simulink model "task_1_scheme"  (R2024a)
settings: Solver=FixedStepAuto  StartTime=0.0  StopTime=5.0  FixedStep=1e-6  RelTol=1e-3
settings Model: Creator=alexe  LastModifiedBy=alexe

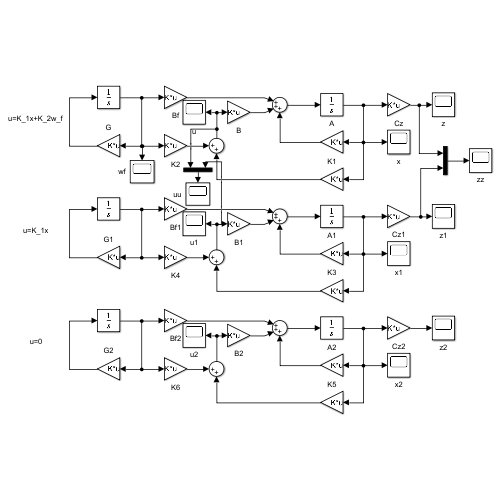
[thumbnail: Simulink's stored preview of the top-level diagram]
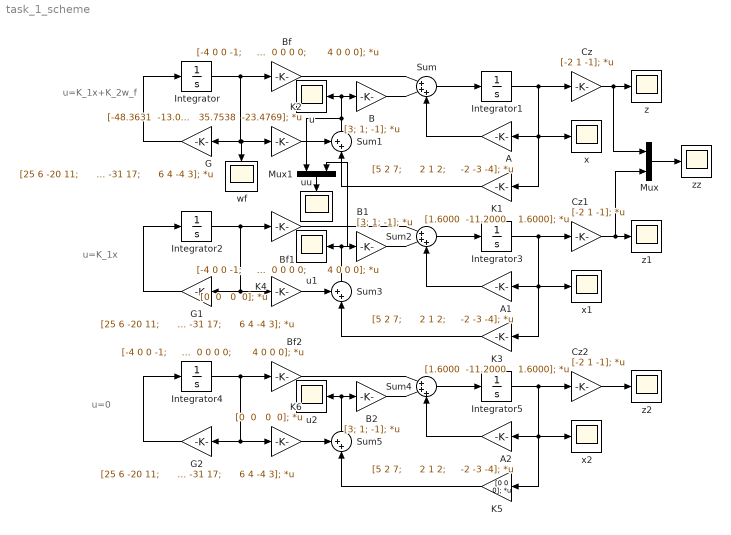
== system task_1_scheme ==
  note: u=K_1x+K_2w_f
  note: u=0
  note: u=K_1x
  A : Gain  Gain=|  Multiplication=Matrix(K*u)
      | [5 2 7;
      |      2 1 2;
      |     -2 -3 -4];
  A1 : Gain  Gain=|  Multiplication=Matrix(K*u)
      | [5 2 7;
      |      2 1 2;
      |     -2 -3 -4];
  A2 : Gain  Gain=|  Multiplication=Matrix(K*u)
      | [5 2 7;
      |      2 1 2;
      |     -2 -3 -4];
  B : Gain  Gain=[3; 1; -1];  Multiplication=Matrix(K*u)
  B1 : Gain  Gain=[3; 1; -1];  Multiplication=Matrix(K*u)
  B2 : Gain  Gain=[3; 1; -1];  Multiplication=Matrix(K*u)
  Bf : Gain  Gain=|  Multiplication=Matrix(K*u)
      | [-4 0 0 -1;
      |       0 0 0 0;
      |       4 0 0 0];
  Bf1 : Gain  Gain=|  Multiplication=Matrix(K*u)
      | [-4 0 0 -1;
      |       0 0 0 0;
      |       4 0 0 0];
  Bf2 : Gain  Gain=|  Multiplication=Matrix(K*u)
      | [-4 0 0 -1;
      |       0 0 0 0;
      |       4 0 0 0];
  Cz : Gain  Gain=[-2 1 -1];  Multiplication=Matrix(K*u)
  Cz1 : Gain  Gain=[-2 1 -1];  Multiplication=Matrix(K*u)
  Cz2 : Gain  Gain=[-2 1 -1];  Multiplication=Matrix(K*u)
  G : Gain  Gain=|  Multiplication=Matrix(K*u)
      | [25 6 -20 11;
      |      14 3 -10 4;
      |      40 11 -31 17;
      |      6 4 -4 3];
  G1 : Gain  Gain=|  Multiplication=Matrix(K*u)
      | [25 6 -20 11;
      |      14 3 -10 4;
      |      40 11 -31 17;
      |      6 4 -4 3];
  G2 : Gain  Gain=|  Multiplication=Matrix(K*u)
      | [25 6 -20 11;
      |      14 3 -10 4;
      |      40 11 -31 17;
      |      6 4 -4 3];
  Integrator : Integrator  InitialCondition=[1;1;1;1]
  Integrator1 : Integrator  InitialCondition=[0;0;0]
  Integrator2 : Integrator  InitialCondition=[1;1;1;1]
  Integrator3 : Integrator  InitialCondition=[0;0;0]
  Integrator4 : Integrator  InitialCondition=[1;1;1;1]
  Integrator5 : Integrator  InitialCondition=[0;0;0]
  K1 : Gain  Gain="[1.6000  -11.2000    1.6000];"  Multiplication=Matrix(K*u)
  K2 : Gain  Gain="[-48.3631  -13.0092   35.7538  -23.4769];"  Multiplication=Matrix(K*u)
  K3 : Gain  Gain="[1.6000  -11.2000    1.6000];"  Multiplication=Matrix(K*u)
  K4 : Gain  Gain="[0  0   0  0];"  Multiplication=Matrix(K*u)
  K5 : Gain  Gain="[0 0  0];"  Multiplication=Matrix(K*u)
  K6 : Gain  Gain="[0  0   0  0];"  Multiplication=Matrix(K*u)
  Mux : Mux  Inputs=2
  Mux1 : Mux  Inputs=2
  Sum : Sum  Inputs=|+++
  Sum1 : Sum  Inputs=++|
  Sum2 : Sum  Inputs=|+++
  Sum3 : Sum  Inputs=++|
  Sum4 : Sum  Inputs=|+++
  Sum5 : Sum  Inputs=++|
  u : Scope
  u1 : Scope
  u2 : Scope
  uu : Scope
  wf : Scope
  x : Scope
  x1 : Scope
  x2 : Scope
  z : Scope
  z1 : Scope
  z2 : Scope
  zz : Scope
  wires:
  G/1 -> Integrator/1
  Integrator/1 -> Bf/1, wf/1, K2/1, G/1
  A/1 -> Sum/3
  Sum/1 -> Integrator1/1
  K1/1 -> Sum1/2
  K2/1 -> Sum1/1
  Sum1/1 -> Mux1/1, u/1, B/1
  Bf/1 -> Sum/1
  B/1 -> Sum/2
  Cz/1 -> Mux/1, z/1
  Integrator1/1 -> Cz/1, x/1, K1/1, A/1
  Bf1/1 -> Sum2/1
  K3/1 -> Sum3/2
  Integrator2/1 -> Bf1/1, K4/1, G1/1
  Sum3/1 -> Mux1/2, u1/1, B1/1
  Integrator3/1 -> Cz1/1, x1/1, K3/1, A1/1
  Sum2/1 -> Integrator3/1
  G1/1 -> Integrator2/1
  K4/1 -> Sum3/1
  A1/1 -> Sum2/3
  B1/1 -> Sum2/2
  Cz1/1 -> Mux/2, z1/1
  Mux/1 -> zz/1
  Bf2/1 -> Sum4/1
  K5/1 -> Sum5/2
  Integrator4/1 -> Bf2/1, K6/1, G2/1
  Sum5/1 -> u2/1, B2/1
  Integrator5/1 -> Cz2/1, x2/1, K5/1, A2/1
  Sum4/1 -> Integrator5/1
  G2/1 -> Integrator4/1
  K6/1 -> Sum5/1
  A2/1 -> Sum4/3
  B2/1 -> Sum4/2
  Cz2/1 -> z2/1
  Mux1/1 -> uu/1
